simulink model "linear_exp_tunable_2026a"  (R2026a)
settings: Solver=FixedStepDiscrete  StopTime=Inf  FixedStep=Ts
model workspace (MAT data in the model file):
  p_active = Simulink.Parameter
  p_active.Value = 0
  p_active.Complexity = 'real'
  p_active.Dimensions = [1 1]
  p_active.DataType = 'auto'
  p_count = Simulink.Parameter
  p_count.Value = 1
  p_count.Complexity = 'real'
  p_count.Dimensions = [1 1]
  p_count.DataType = 'auto'
  p_ff = Simulink.Parameter
  p_ff.Value = [0 0 0 0 0 0 0 0 0 0 0 0 ... (131072 elements, 131072x1)]
  p_ff.Complexity = 'real'
  p_ff.Dimensions = [131072 1]
  p_ff.CoderInfo.StorageClass = 'ImportedExtern'
  p_ff.DataType = 'auto'
  p_ref = Simulink.Parameter
  p_ref.Value = [0 0 0 0 0 0 0 0 0 0 0 0 ... (131072 elements, 131072x1)]
  p_ref.Complexity = 'real'
  p_ref.Dimensions = [131072 1]
  p_ref.CoderInfo.StorageClass = 'ImportedExtern'
  p_ref.DataType = 'auto'
  p_servo = Simulink.Parameter
  p_servo.Value = 0
  p_servo.Complexity = 'real'
  p_servo.Dimensions = [1 1]
  p_servo.DataType = 'auto'
  servo_switch = Simulink.Parameter
  servo_switch.Value = 1
  servo_switch.Complexity = 'real'
  servo_switch.Dimensions = [1 1]
  servo_switch.DataType = 'auto'
undefined symbols (not defined in the file): CURRENT_TO_UNIT, ENCODER_RESOLUTION, feedbackFlag, MAX_INPUT, set_ref, Ts, TwinCAT
libraries: TcTargetLib x5, cstblocks_lti x1, simulink x1
settings Model: SimulationMode=external  Creator=AKZW  LastModifiedBy=AKZW
settings OptimizationCC: LocalBlockOutputs=off
settings DebuggingCC: InheritedTsInSrcMsg=none
settings SFSimCC: UsePrecompiledLibraries=Avoid
settings RTWCC: SystemTargetFile=TwinCatGrt.tlc  GenCodeOnly=on  GenerateMakefile=off  TemplateMakefile=tcgrt_msbuild.tmf  CustomHeaderCode="#include \"linear_exp_tunable_2025a_parameters.h\""  CustomSource=src/linear_exp_tunable_2025a_parameters.cpp  TargetLang=C++  Description=TwinCAT GRT Target
settings STFCustomTargetCC: SystemTargetFile=TwinCatGrt.tlc  TargetLangStandard=C++11 (ISO)  MultiwordLength=2048.0  ConcurrentExecutionCompliant=on  CombineOutputUpdateFcns=on  MatFileLogging=on  CPPClassGenCompliant=on  GRTInterface=off  TcProject_Generate=on  TcProject_PlcVarPrefixes=PVOID=p | BOOL=b | BOOL32=b | DATE=d | TIME_OF_DATE=td | TIME=t | LTIME=t | GUID=n  TcProject_Versioning=Versioned  TcProject_ClassFactoryName=$<Project:Name>  TcProject_LowestCompatibleTcBuild=$<TwinCAT:Version:BUILD>  TcCom_OnlineChangeRestoreDataAreas=off  TcProject_VendorIcon=$<TE140x:Icon>  TcProject_ProductName=$<ModuleGenerator:ProductId> $<ModuleGenerator:Version:MAJOR.MINOR>  TcProject_VersionSrc=$<LatestTMFile>  TcProject_Copyright=Copyright $<VendorName> $<LocalDateTime:%Y>  TcProject_Description=TwinCAT executable file, generated by TwinCAT $<ModuleGenerator:ProductId>  TcProject_VendorName=TE140x Module Vendor  TcProject_IncrementVersion=Revision  TcProject_DrvFileVersion=$<VersionFromFile>  TcProject_DrvProductVersion=$<DrvFileVersion>  TcProject_CreateScopedEnums=Auto  TcProject_UseDataExchangeModules=off  TcProject_MaxVisibleArrayElements=200U  TcProject_CreateUniqueEnumItemNames=off  TcProject_UseIntrinsics=on  TcCom_OemLicenses=$<Project:OemLicenses>  TcProject_DataExchangeModulesVersion=$<ModuleGenerator:DataExchange:Version>  TcProject_UseCodeDescriptor=on  TcProject_CoderCppNamespace=coder  TcCom_ModuleCaller=CyclicTask  TcProject_PreferIntOverLong=off  TcProject_UseStaticStlString=off  TcCom_StepSizeAdaptation=RequireMatchingTaskCycleTime  TcProject_StaticStlStringCapacity=Auto  TcProject_IgnorePseudoArrayDimensions=off  TcCom_ExecuteModelCode=on  TcProject_UseCodeInfoExporter=on  TcProject_PreferToolArchitectureX64=on  TcProject_UseNativeBlockDiagramExport=off  TcCom_ResolveMaskedSubsystems=on  TcProject_UseDescriptorCodeType=on  TcProject_UseLLVMCodeInfo=on  TcProject_BuildSystem=Auto  TcProject_EnableNewPlatforms=off  TcProject_CppLanguageStandard=Default  TcCom_BlockDiagramDebugInfoExport=on  TcProject_CLanguageStandard=Default  TcProject_Verbosity=Normal  TcProject_PublishPlatformtoolset=Auto  TcProject_Publish=on  TcProject_PublishTcOSx64E=off  TcProject_PublishConfiguration=Release  TcCom_OutputDataAccess=Output Source DataArea  TcProject_PublishTcRTx86=on  TcProject_PublishTcRTx64=on  TcProject_PublishTcOSx64=off  TcProject_PublishTcUMx64=off  TcProject_PublishTcOSARMv8A=off  TcProject_PublishTcOSARMv7A=off  TcProject_PublishTcOSARMv7M=off  TcProject_PublishTcUMx86=off  TcProject_SignWithTwinCatCertificate=inherit default  TcProject_ForceRebuildForPublish=off  TcCom_ParametersDataAccess=Internal DataArea  TcProject_PublishParallel=on  TcProject_BuildWithWdk=inherit default  TcCom_ParametersReadOnly=off  TcProject_UseTmxExtension=Auto  TcProject_SignTwinCatCertName=TcTestCert  TcCom_BlockIoDataAccess=Internal DataArea  TcProject_TmxInstall=on  TcCom_ContStateDataAccess=Internal DataArea  TcProject_GenerateVsSolution=No  TcCom_ContStateReadOnly=on  TcProject_DeployRestart=off  TcProject_PreCodeGenerationCallbackFcn=compact_tunable_trajectory_tlc_export  TcCom_DWorkReadOnly=on  TcCom_DataStoreDataAccess=None  TcProject_LibCatPath=$<Project:Dir>\$<Project:Name>.libcat.xml  TcProject_LibraryCategories=$<VendorName>  TcCom_DataStoreReadOnly=off  TcCom_AllowDataAreaForSharedData=off  TcProject_GeneratePlcLibrary=off  TcProject_InstallPlcLibrary=off  TcProject_GenerateStructDutsWithDefaultValues=Auto  TcCom_OriginalIoBlockNames=off  TcCom_Generate=on  TcCom_StrictAccessLock=on  TcCom_OnlineChange=off  TcCom_Legacy_ModuleBuildInfoParam=on  TcPlcFb_Generate=off  TcCom_GroupName=TE140x|Simulink Modules  TcCom_GroupDisplayName=$<GroupName>  TcPlcFb_InitExceptionHandling=CallerExceptions  TcCom_GroupIcon=$<TE140x:Icon>  TcCom_ModuleIcon=$<TE140x:Icon>  TcCom_InitExceptionHandling=CallerExceptions  TcCom_UpdateExceptionHandling=CallerExceptions  TcCom_TcComWrapperFb=off  TcCom_TcComWrapperFbProperties=off  TcCom_TcComWrapperFbPropertyMonitoring=NoMonitoring  TcCom_CallerVerification=Default  TcCom_ExecutionSequence=UpdateBeforeOutputMapping  TcCom_BlockDiagramExport=on  TcCom_ExtendSignalResolution=off  TcCom_BlockDiagramVariableAccess=AssignToParent  TcCom_ExecutionInfoParam=on  TcCom_ExecutionInfoOutput=off  TcCom_MonitorExecutionTime=off  TcCom_AccessLockState=Auto  TcCom_InputDataAccess=Input Destination DataArea  TcCom_InputCreateSymbols=on  TcCom_InputReadOnly=off  TcCom_InputInitValues=off  TcCom_OutputCreateSymbols=on  TcCom_OutputReadOnly=on  TcCom_ParametersCreateSymbols=on  TcCom_ParametersInitValues=off  TcCom_GlobalParamDefaultSharing=Define  TcCom_BlockIoCreateSymbols=on  TcCom_BlockIoReadOnly=on  TcCom_ContStateCreateSymbols=on  TcCom_DWorkDataAccess=Internal DataArea  TcCom_DWorkCreateSymbols=on  TcCom_DataStoreCreateSymbols=on  TcCom_MaxInternalDataAreaParts=5U  TcCom_VariableSymbolMapping=Identical  TcCom_VariableSymbolMappingCustom=$<ModelName>_U=Input|$<ModelName>_Y=Output|$<ModelName>_P=ModelParameters|$<ModelName>_B=BlockIO|$<ModelName>_DW=DWork|$<ModelName>_X=ContStates  TcCom_ExtModeRtAllowExecutionCommands=on  TcCom_ExtModeRtWaitForStart=on  TcCom_ExtModeRtAllowForParameterChange=on  TcPlcFb_UpdateExceptionHandling=CallerExceptions  TcPlcFb_OemLicenses=$<Project:OemLicenses>  TcPlcFb_MonitorExecutionTime=off  TcPlcFb_ExtModeRtAllowExecutionCommands=off  TcPlcFb_ExtModeRtWaitForStart=off  TcPlcFb_ExtModeRtAllowForParameterChange=off
settings GRTTargetCC: ExtMode=on  ExtModeMexFile=TcExtModeClient  TargetLangStandard=C++11 (ISO)  ParMdlRefBuildCompliant=off  CompOptLevelCompliant=off

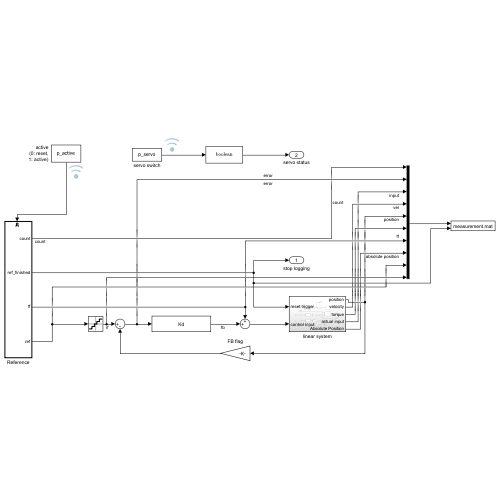
[thumbnail: Simulink's stored preview of the top-level diagram]
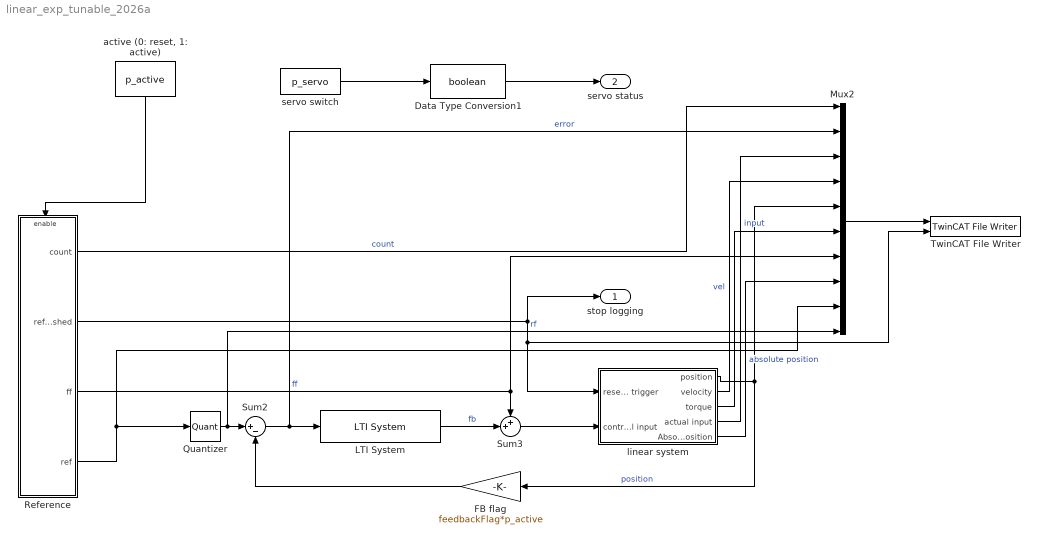
== system linear_exp_tunable_2026a ==
  Data Type Conversion1 : DataTypeConversion  OutDataTypeStr=boolean  SaturateOnIntegerOverflow=off  RndMeth=Floor
  FB flag : Gain  Gain=feedbackFlag*p_active
  LTI System : cstblocks_lti/LTI System  sys=Kd  IC=[]  PadeOrder=0
  Mux2 : Mux  Inputs=10
  Quantizer : Quantizer  QuantizationInterval=ENCODER_RESOLUTION
  Reference : Subsystem  TreatAsAtomicUnit=on
  Sum2 : Sum  Inputs=|+-
  Sum3 : Sum  Inputs=++|
  TwinCAT File Writer : TcTargetLib/TwinCAT File Writer  PortDataType=double  PortDim=-1  SampleTime=-1  MatFileName=C:\expdata\measurement.mat  MaxFileByteSize=0  MaxFileCount=0  Pause=on  TraceMode=3  WriteTimestamp=on  PauseAsInput=on  CloseOnPause=on
      settings: SourceProductName=Beckhoff TwinCAT Target
  "active (0: reset, 1: active)" : Constant  Value=p_active  SampleTime=Ts
  linear system : Subsystem
  servo switch : Constant  Value=p_servo  SampleTime=Ts
  stop logging : Outport  VectorParamsAs1DForOutWhenUnconnected=off
  servo status : Outport  Port=2
  wires:
  Quantizer/1 -> Mux2/10, Sum2/1  "rf"
  Sum3/1 -> linear system/2(control input)
  Reference/3(ff) -> Sum3/1, Mux2/7  "ff"
  FB flag/1 -> Sum2/2
  Sum2/1 -> Mux2/2, LTI System/1  "error"
  linear system/5(Absolute Position) -> Mux2/8  "absolute position"
  Data Type Conversion1/1 -> servo status/1
  "active (0: reset, 1: active)"/1 -> Reference/Enable
  linear system/4(actual input) -> Mux2/3  "input"
  Reference/4(ref) -> Mux2/9, Quantizer/1
  linear system/3(torque) -> Mux2/6
  linear system/2(velocity) -> Mux2/4  "vel"
  LTI System/1 -> Sum3/2  "fb"
  Reference/2(ref_finished) -> stop logging/1, linear system/1(reset trigger), TwinCAT File Writer/2
  Reference/1(count) -> Mux2/1  "count"
  servo switch/1 -> Data Type Conversion1/1
  linear system/1(position) -> FB flag/1, Mux2/5  "position"
  Mux2/1 -> TwinCAT File Writer/1

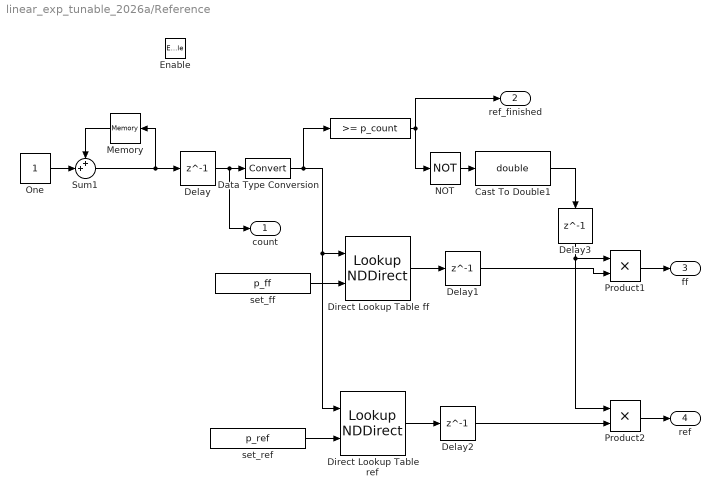
== system linear_exp_tunable_2026a/Reference ==
  Enable : EnablePort  StatesWhenEnabling=reset
  " " : simulink/Logic and Bit Operations/Compare To Constant  relop=>=  const=p_count  OutDataTypeStr=boolean
  Cast To Double1 : DataTypeConversion  OutDataTypeStr=double  SaturateOnIntegerOverflow=off  RndMeth=Floor
  Data Type Conversion : DataTypeConversion  SaturateOnIntegerOverflow=off  RndMeth=Floor
  Delay{,1..3} (4 alike) : Delay  DelayLength=1
  Direct Lookup Table ff : LookupNDDirect  NumberOfTableDimensions=1  TableIsInput=on  Table=[4 5 ;16 19 ]
  Direct Lookup Table ref : LookupNDDirect  NumberOfTableDimensions=1  TableIsInput=on  Table=set_ref  TableDataTypeStr=fixdt('double', 'DataTypeOverride', 'Off')
  Memory : Memory
  NOT : Logic  Operator=NOT  IconShape=distinctive  AllPortsSameDT=off  OutDataTypeStr=boolean
  One : Constant  OutDataTypeStr=Inherit: Inherit via back propagation
  Product1 : Product
  Product2 : Product
  Sum1 : Sum  Inputs=++|
  set_ff : Constant  Value=p_ff  SampleTime=Ts
  set_ref : Constant  Value=p_ref  OutDataTypeStr=fixdt('double', 'DataTypeOverride', 'Off')  SampleTime=Ts
  count : Outport
  ref_finished : Outport  Port=2  InitialOutput=true
  ff : Outport  Port=3  OutputWhenDisabled=reset  InitialOutput=0
  ref : Outport  Port=4  OutputWhenDisabled=reset  InitialOutput=0
  wires:
  Delay1/1 -> Product1/2
  Delay/1 -> count/1, Data Type Conversion/1
  set_ff/1 -> Direct Lookup Table ff/2
  NOT/1 -> Cast To Double1/1
  Cast To Double1/1 -> Delay3/1
  " "/1 -> ref_finished/1, NOT/1
  Direct Lookup Table ff/1 -> Delay1/1
  Direct Lookup Table ref/1 -> Delay2/1
  Delay2/1 -> Product2/2
  set_ref/1 -> Direct Lookup Table ref/2
  Sum1/1 -> Delay/1, Memory/1
  Data Type Conversion/1 -> Direct Lookup Table ref/1, Direct Lookup Table ff/1, " "/1
  Delay3/1 -> Product2/1, Product1/1
  Memory/1 -> Sum1/1
  One/1 -> Sum1/2
  Product1/1 -> ff/1
  Product2/1 -> ref/1

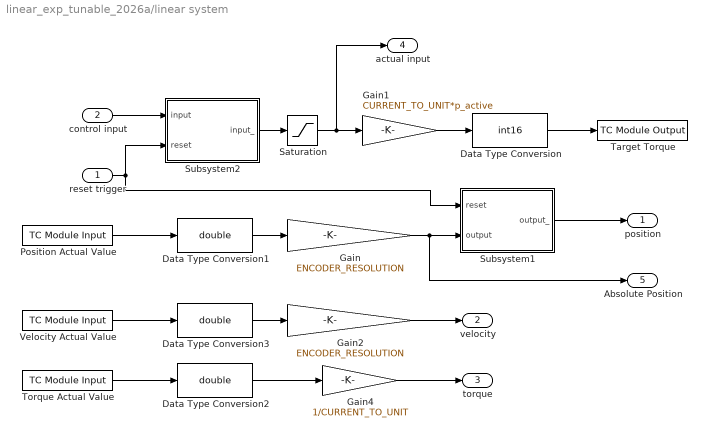
== system linear_exp_tunable_2026a/linear system ==
  reset trigger : Inport
  control input : Inport  Port=2
  Data Type Conversion : DataTypeConversion  OutDataTypeStr=int16  SaturateOnIntegerOverflow=off  RndMeth=Floor
  Data Type Conversion1 : DataTypeConversion  OutDataTypeStr=double  SaturateOnIntegerOverflow=off  RndMeth=Floor
  Data Type Conversion2 : DataTypeConversion  OutDataTypeStr=double  SaturateOnIntegerOverflow=off  RndMeth=Floor
  Data Type Conversion3 : DataTypeConversion  OutDataTypeStr=double  SaturateOnIntegerOverflow=off  RndMeth=Floor
  Gain : Gain  Gain=ENCODER_RESOLUTION
  Gain1 : Gain  Gain=CURRENT_TO_UNIT*p_active
  Gain2 : Gain  Gain=ENCODER_RESOLUTION
  Gain4 : Gain  Gain=1/CURRENT_TO_UNIT
  Position Actual Value : TcTargetLib/TC Module Input  PortDataType=int32  Value=0  SampleTime=-1  PortDim=-1  PortComplexity=auto  SymbolName=TwinCAT.ModuleGenerator.Simulink.BlockPathToSymbolName(gcb,true)  CodeGenConnectType=DataArea (InputDst)  DataTypeOverride=off
      settings: SourceProductName=Beckhoff TwinCAT Target
  Saturation : Saturate  UpperLimit=MAX_INPUT  LowerLimit=-MAX_INPUT
  Subsystem1 : Subsystem
  Subsystem2 : Subsystem
  Target Torque : TcTargetLib/TC Module Output  PortDataType=Inherit: auto  SampleTime=-1  PortDim=-1  PortComplexity=auto  SymbolName=TwinCAT.ModuleGenerator.Simulink.BlockPathToSymbolName(gcb,true)  CodeGenConnectType=DataArea (OutputSrc)  DataTypeOverride=off
      settings: SourceProductName=Beckhoff TwinCAT Target
  Torque Actual Value : TcTargetLib/TC Module Input  PortDataType=int16  Value=0  SampleTime=-1  PortDim=-1  PortComplexity=auto  SymbolName=TwinCAT.ModuleGenerator.Simulink.BlockPathToSymbolName(gcb,true)  CodeGenConnectType=DataArea (InputDst)  DataTypeOverride=off
      settings: SourceProductName=Beckhoff TwinCAT Target
  Velocity Actual Value : TcTargetLib/TC Module Input  PortDataType=int32  Value=0  SampleTime=-1  PortDim=-1  PortComplexity=auto  SymbolName=TwinCAT.ModuleGenerator.Simulink.BlockPathToSymbolName(gcb,true)  CodeGenConnectType=DataArea (InputDst)  DataTypeOverride=off
      settings: SourceProductName=Beckhoff TwinCAT Target
  position : Outport  VectorParamsAs1DForOutWhenUnconnected=off
  velocity : Outport  Port=2  VectorParamsAs1DForOutWhenUnconnected=off
  torque : Outport  Port=3  VectorParamsAs1DForOutWhenUnconnected=off
  actual input : Outport  Port=4  VectorParamsAs1DForOutWhenUnconnected=off
  Absolute Position : Outport  Port=5  VectorParamsAs1DForOutWhenUnconnected=off
  wires:
  Gain1/1 -> Data Type Conversion/1
  Data Type Conversion1/1 -> Gain/1
  Gain/1 -> Absolute Position/1, Subsystem1/2(output)
  Gain2/1 -> velocity/1
  Velocity Actual Value/1 -> Data Type Conversion3/1
  Position Actual Value/1 -> Data Type Conversion1/1
  Data Type Conversion3/1 -> Gain2/1
  Data Type Conversion/1 -> Target Torque/1
  control input/1 -> Subsystem2/1(input)
  Subsystem1/1(output_) -> position/1
  Subsystem2/1(input_) -> Saturation/1
  Saturation/1 -> actual input/1, Gain1/1
  reset trigger/1 -> Subsystem1/1(reset), Subsystem2/2(reset)
  Torque Actual Value/1 -> Data Type Conversion2/1
  Data Type Conversion2/1 -> Gain4/1
  Gain4/1 -> torque/1

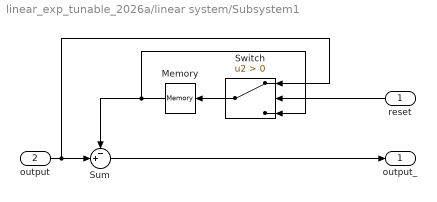
== system linear_exp_tunable_2026a/linear system/Subsystem1 ==
  reset : Inport
  output : Inport  Port=2
  Memory : Memory
  Sum : Sum  Inputs=-+|
  Switch : Switch  Criteria=u2 > Threshold  SaturateOnIntegerOverflow=off  InputSameDT=off
  output_ : Outport  VectorParamsAs1DForOutWhenUnconnected=off
  wires:
  reset/1 -> Switch/2
  Sum/1 -> output_/1
  output/1 -> Sum/2, Switch/1
  Switch/1 -> Memory/1
  Memory/1 -> Sum/1, Switch/3

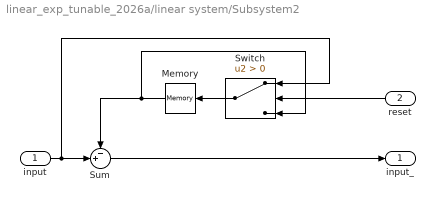
== system linear_exp_tunable_2026a/linear system/Subsystem2 ==
  input : Inport
  reset : Inport  Port=2
  Memory : Memory
  Sum : Sum  Inputs=-+|
  Switch : Switch  Criteria=u2 > Threshold  SaturateOnIntegerOverflow=off  InputSameDT=off
  input_ : Outport  VectorParamsAs1DForOutWhenUnconnected=off
  wires:
  Memory/1 -> Switch/3, Sum/1
  Switch/1 -> Memory/1
  input/1 -> Switch/1, Sum/2
  Sum/1 -> input_/1
  reset/1 -> Switch/2
